simulink model "aerotest"  (R2021b)
settings: Solver=VariableStepAuto  StartTime=0.0  StopTime=10.0  RelTol=1e-3
undefined symbols (not defined in the file or in its folder): admireDB
libraries: simulink_extras x103, simulink x24, aerolibatmos2 x1
(part 1 of 13)
settings Model: Creator=mehme  LastModifiedBy=mehme

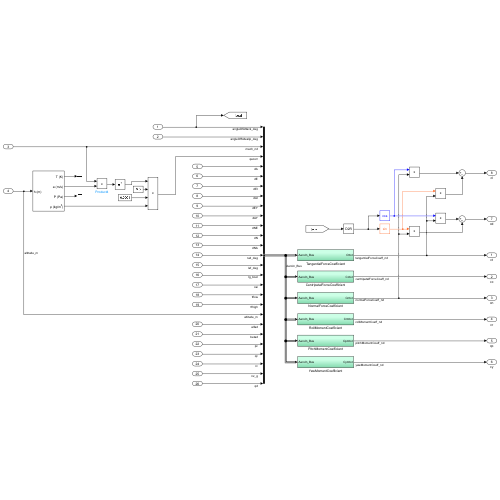
[thumbnail: Simulink's stored preview of the top-level diagram]
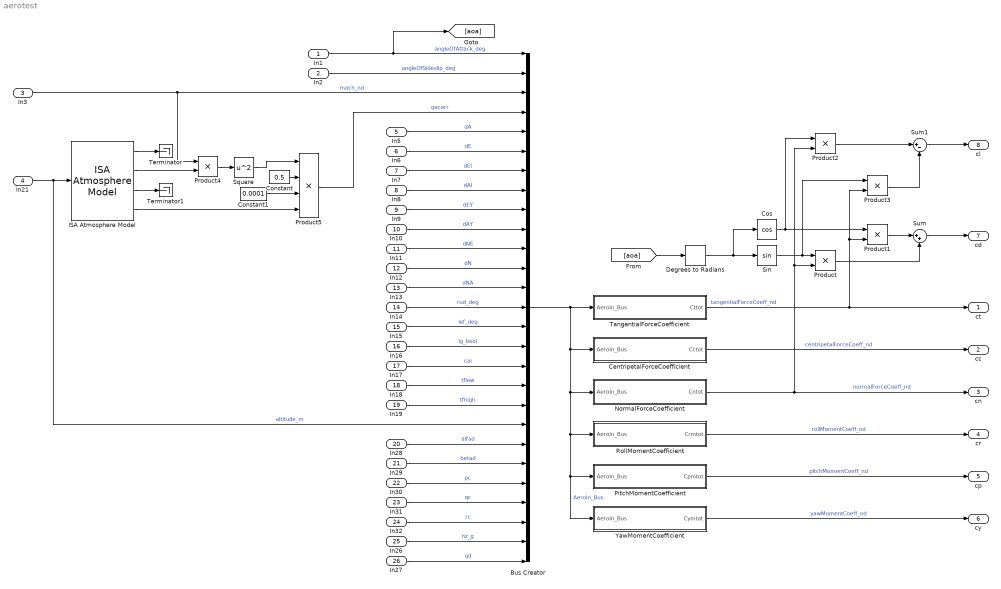
== system aerotest ==
  In1 : Inport
  In2 : Inport  Port=2
  In3 : Inport  Port=3
  In21 : Inport  Port=4
  In5 : Inport  Port=5
  In6 : Inport  Port=6
  In7 : Inport  Port=7
  In8 : Inport  Port=8
  In9 : Inport  Port=9
  In10 : Inport  Port=10
  In11 : Inport  Port=11
  In12 : Inport  Port=12
  In13 : Inport  Port=13
  In14 : Inport  Port=14
  In15 : Inport  Port=15
  In16 : Inport  Port=16
  In17 : Inport  Port=17
  In18 : Inport  Port=18
  In19 : Inport  Port=19
  In28 : Inport  Port=20
  In29 : Inport  Port=21
  In30 : Inport  Port=22
  In31 : Inport  Port=23
  In32 : Inport  Port=24
  In26 : Inport  Port=25
  In27 : Inport  Port=26
  Bus Creator : BusCreator  Inputs=27
  CentripetalForceCoefficient : Subsystem
  Constant : Constant  Value=0.5
  Constant1 : Constant  Value=0.0001
  Cos : Trigonometry  Operator=cos
  Degrees to Radians : simulink_extras/Transformations/Degrees to Radians
  ISA Atmosphere Model : aerolibatmos2/ISA Atmosphere Model  custom=off  g=9.80665  gamma=1.4  R=287.0531  L=0.0065  h_trop=11000  h_strat=20000  rho0=1.225  P0=101325  T0=288.15  h0=0
  NormalForceCoefficient : Subsystem
  PitchMomentCoefficient : Subsystem
  Product{,1..4} (5 alike) : Product
  Product5 : Product  Inputs=4
  RollMomentCoefficient : Subsystem
  Sin : Trigonometry
  Square : Math  Operator=square  SaturateOnIntegerOverflow=on
  Sum : Sum  Inputs=|++
  Sum1 : Sum  Inputs=|+-
  TangentialForceCoefficient : Subsystem
  Terminator : Terminator
  Terminator1 : Terminator
  YawMomentCoefficient : Subsystem
  ct : Outport
  cc : Outport  Port=2
  cn : Outport  Port=3
  cr : Outport  Port=4
  cp : Outport  Port=5
  cy : Outport  Port=6
  cd : Outport  Port=7
  cl : Outport  Port=8
  wires:
  Bus Creator/1 -> TangentialForceCoefficient/1(AeroIn_Bus), CentripetalForceCoefficient/1(AeroIn_Bus), NormalForceCoefficient/1(AeroIn_Bus), RollMomentCoefficient/1(AeroIn_Bus), YawMomentCoefficient/1(AeroIn_Bus), PitchMomentCoefficient/1(AeroIn_Bus)  "AeroIn_Bus"
  CentripetalForceCoefficient/1(Cctot) -> cc/1  "centripetalForceCoeff_nd"
  TangentialForceCoefficient/1(Cttot) -> Product3/2, Product1/2, ct/1  "tangentialForceCoeff_nd"
  NormalForceCoefficient/1(Cntot) -> cn/1, Product2/2, Product/2  "normalForceCoeff_nd"
  YawMomentCoefficient/1(Cymtot) -> cy/1  "yawMomentCoeff_nd"
  RollMomentCoefficient/1(Crmtot) -> cr/1  "rollMomentCoeff_nd"
  PitchMomentCoefficient/1(Cpmtot) -> cp/1  "pitchMomentCoeff_nd"
  In10/1 -> Bus Creator/10  "dAY"
  In16/1 -> Bus Creator/16  "lg_bool"
  In26/1 -> Bus Creator/26  "nz_g"
  In18/1 -> Bus Creator/18  "tflow"
  In14/1 -> Bus Creator/14  "rud_deg"
  In31/1 -> Bus Creator/24  "qc"
  In30/1 -> Bus Creator/23  "pc"
  In28/1 -> Bus Creator/21  "alfad"
  In15/1 -> Bus Creator/15  "lef_deg"
  In7/1 -> Bus Creator/7  "dEI"
  In13/1 -> Bus Creator/13  "dNA"
  In11/1 -> Bus Creator/11  "dNE"
  In21/1 -> Bus Creator/20, ISA Atmosphere Model/1  "altitude_m"
  In8/1 -> Bus Creator/8  "dAI"
  In17/1 -> Bus Creator/17  "cai"
  In5/1 -> Bus Creator/5  "dA"
  In9/1 -> Bus Creator/9  "dEY"
  In19/1 -> Bus Creator/19  "tfhigh"
  In6/1 -> Bus Creator/6  "dE"
  In2/1 -> Bus Creator/2  "angleOfSideslip_deg"
  Product5/1 -> Bus Creator/4  "qacorr"
  In27/1 -> Bus Creator/27  "qd"
  In3/1 -> Bus Creator/3, Product4/1  "mach_nd"
  In12/1 -> Bus Creator/12  "dN"
  In1/1 -> Bus Creator/1, [aoa]  "angleOfAttack_deg"
  In29/1 -> Bus Creator/22  "betad"
  In32/1 -> Bus Creator/25  "rc"
  Degrees to Radians/1 -> Cos/1, Sin/1
  Sin/1 -> Product3/1, Product/1
  Cos/1 -> Product2/1, Product1/1
  Product1/1 -> Sum/1
  Product/1 -> Sum/2
  Product2/1 -> Sum1/1
  Product3/1 -> Sum1/2
  Sum/1 -> cd/1
  Sum1/1 -> cl/1
  ISA Atmosphere Model/1 -> Terminator/1
  ISA Atmosphere Model/3 -> Terminator1/1
  ISA Atmosphere Model/2 -> Product4/2
  Product4/1 -> Square/1
  Square/1 -> Product5/1
  ISA Atmosphere Model/4 -> Product5/4
  Constant/1 -> Product5/2
  Constant1/1 -> Product5/3
  [aoa] -> Degrees to Radians/1

== system aerotest/CentripetalForceCoefficient ==
  AeroIn_Bus : Inport
  Bus Selector : BusSelector  OutputSignals=mach_nd
  MachRegion1 : Subsystem
  MachRegion2 : Subsystem
  MachRegion3 : Subsystem
  MachRegion4 : Subsystem
  Subsystem : Subsystem
  Cctot : Outport
  wires:
  Subsystem/1(Cctot) -> Cctot/1
  MachRegion3/1(cctot) -> Subsystem/4(CctotMR3)
  MachRegion2/1(cctot) -> Subsystem/3(CctotMR2)
  MachRegion4/1(cttot) -> Subsystem/5(CctotMR4)
  Bus Selector/1 -> Subsystem/1(mach_nd)  "<mach_nd>"
  AeroIn_Bus/1 -> MachRegion2/1(AeroIn_Bus), MachRegion3/1(AeroIn_Bus), MachRegion4/1(AeroIn_Bus), MachRegion1/1(AeroIn_Bus), Bus Selector/1
  MachRegion1/1(cctot) -> Subsystem/2(CctotMR1)

== system aerotest/NormalForceCoefficient ==
  AeroIn_Bus : Inport
  Bus Selector : BusSelector  OutputSignals=mach_nd
  MachRegion1 : Subsystem
  MachRegion2 : Subsystem
  MachRegion3 : Subsystem
  Subsystem : Subsystem
  Cntot : Outport
  wires:
  Subsystem/1(Cntot) -> Cntot/1
  Bus Selector/1 -> Subsystem/1(mach_nd)  "<mach_nd>"
  MachRegion2/1(Cntot) -> Subsystem/3(CntotMR2)
  AeroIn_Bus/1 -> MachRegion2/1(Misc_Bus), MachRegion3/1(Misc_Bus), MachRegion1/1(Misc_Bus), Bus Selector/1
  MachRegion3/1(Cntot) -> Subsystem/4(CntotMR3)
  MachRegion1/1(Cntot) -> Subsystem/2(CntotMR1)

== system aerotest/PitchMomentCoefficient ==
  AeroIn_Bus : Inport
  Bus Selector : BusSelector  OutputSignals=mach_nd
  MachRegion1 : Subsystem
  MachRegion2 : Subsystem
  MachRegion3 : Subsystem
  Subsystem : Subsystem
  Cpmtot : Outport
  wires:
  Subsystem/1(Cpmtot) -> Cpmtot/1
  MachRegion1/1(Cpmtot) -> Subsystem/2(CpmtotMR1)
  MachRegion2/1(Cpmtot) -> Subsystem/3(CpmtotMR2)
  MachRegion3/1(Cpmtot) -> Subsystem/4(CpmtotMR3)
  AeroIn_Bus/1 -> MachRegion2/1(Misc_Bus), MachRegion3/1(Misc_Bus), MachRegion1/1(Misc_Bus), Bus Selector/1
  Bus Selector/1 -> Subsystem/1(mach_nd)  "<mach_nd>"

== system aerotest/RollMomentCoefficient ==
  AeroIn_Bus : Inport
  Bus Selector : BusSelector  OutputSignals=mach_nd
  MachRegion1 : Subsystem
  MachRegion2 : Subsystem
  MachRegion3 : Subsystem
  MachRegion4 : Subsystem
  Subsystem : Subsystem
  Crmtot : Outport
  wires:
  Subsystem/1(Crmtot) -> Crmtot/1
  MachRegion4/1(crmtot) -> Subsystem/5(CrmtotMR4)
  MachRegion3/1(crmtot) -> Subsystem/4(CrmtotMR3)
  MachRegion2/1(crmtot) -> Subsystem/3(CrmtotMR2)
  MachRegion1/1(crmtot) -> Subsystem/2(CrmtotMR1)
  Bus Selector/1 -> Subsystem/1(mach_nd)  "<mach_nd>"
  AeroIn_Bus/1 -> MachRegion1/1(AeroIn_Bus), Bus Selector/1, MachRegion2/1(AeroIn_Bus), MachRegion3/1(AeroIn_Bus), MachRegion4/1(AeroIn_Bus)

== system aerotest/TangentialForceCoefficient ==
  AeroIn_Bus : Inport
  Bus Selector : BusSelector  OutputSignals=mach_nd
  MachRegion1 : Subsystem
  MachRegion2 : Subsystem
  MachRegion3 : Subsystem
  Subsystem : Subsystem
  Cttot : Outport
  wires:
  Subsystem/1(Out1) -> Cttot/1
  MachRegion3/1(cttotMR3) -> Subsystem/4(cttotMR3)
  MachRegion2/1(cttotMR2) -> Subsystem/3(cttotMR2)
  MachRegion1/1(cttotMR1) -> Subsystem/2(cttotMR1)
  Bus Selector/1 -> Subsystem/1(mach_nd)  "<mach_nd>"
  AeroIn_Bus/1 -> MachRegion1/1(AeroIn_Bus), MachRegion2/1(AeroIn_Bus), MachRegion3/1(AeroIn_Bus), Bus Selector/1  "AeroIn_Bus"

== system aerotest/YawMomentCoefficient ==
  AeroIn_Bus : Inport
  Bus Selector : BusSelector  OutputSignals=mach_nd
  MachRegion1 : Subsystem
  MachRegion2 : Subsystem
  MachRegion3 : Subsystem
  MachRegion4 : Subsystem
  Subsystem : Subsystem
  Cymtot : Outport
  wires:
  Subsystem/1(Cymtot) -> Cymtot/1
  Bus Selector/1 -> Subsystem/1(mach_nd)  "<mach_nd>"
  MachRegion1/1(Cymtot) -> Subsystem/2(CymtotMR1)
  MachRegion3/1(Cymtot) -> Subsystem/4(CymtotMR3)
  AeroIn_Bus/1 -> MachRegion1/1(AeroIn_Bus), Bus Selector/1, MachRegion2/1(AeroIn_Bus), MachRegion3/1(AeroIn_Bus), MachRegion4/1(AeroIn_Bus)
  MachRegion4/1(Cymtot) -> Subsystem/5(CymtotMR4)
  MachRegion2/1(Cymtot) -> Subsystem/3(CymtotMR2)

== system aerotest/CentripetalForceCoefficient/MachRegion1 ==
  note: Mach <= 0.4
  AeroIn_Bus : Inport
  Bus Creator : BusCreator  Inputs=3
  Ccbcai : Subsystem
  Ccbde : Subsystem
  Ccbdle : Subsystem
  Ccbdn : Subsystem
  Ccbeta : Subsystem
  Ccbetad : Subsystem
  Ccblg : Subsystem
  Ccdai : Subsystem
  Ccdaib : Subsystem
  Ccday : Subsystem
  Ccdayb : Subsystem
  Ccdna : Subsystem
  Ccdr : Subsystem
  Ccp : Subsystem
  Ccpbeta : Subsystem
  Ccr : Subsystem
  Ccrbeta : Subsystem
  Sum : Sum  Inputs=17
  eoeff1 : Subsystem
  cctot : Outport
  wires:
  Ccrbeta/1(Ccrbeta) -> Sum/17  "Ccrbeta"
  Ccr/1(Ccr) -> Sum/16  "Ccr"
  Ccpbeta/1(Ccpbeta) -> Sum/15  "Ccpbeta"
  Ccp/1(Ccp) -> Sum/14  "Ccp"
  Ccbetad/1(Ccbetad) -> Sum/13  "Ccbetad"
  Ccdna/1(Ccdna) -> Sum/12  "Ccdna"
  Ccdayb/1(Ccdayb) -> Sum/11  "Ccdayb"
  Ccday/1(Ccday) -> Sum/10  "Ccday"
  Ccdaib/1(Ccdaib) -> Sum/9  "Ccdaib"
  Ccdai/1(Ccdai) -> Sum/8  "Ccdai"
  Ccdr/1(Ccdr) -> Sum/7  "Ccdr"
  Ccbcai/1(Ccbcai) -> Sum/6  "Ccbcai"
  Ccbdle/1(Ccbdle) -> Sum/5  "Ccbdle"
  Ccbdn/1(Ccbdn) -> Sum/4  "Ccbdn"
  Ccbde/1(Ccbde) -> Sum/3  "Ccbde"
  Ccblg/1(Ccblg) -> Sum/2  "Ccblg"
  Ccbeta/1(Ccbeta) -> Sum/1  "Ccbeta"
  Bus Creator/1 -> Ccp/1(in_bus), Ccpbeta/1(in_bus), Ccr/1(in_bus), Ccrbeta/1(in_bus), Ccbetad/1(in_bus), Ccdna/1(in_bus), Ccdayb/1(in_bus), Ccday/1(in_bus), Ccdaib/1(in_bus), Ccdai/1(in_bus), Ccdr/1(in_bus), Ccbcai/1(in_bus), Ccbdle/1(in_bus), Ccbdn/1(in_bus), Ccbde/1(in_bus), Ccblg/1(in_bus), Ccbeta/1(in_bus)  "in_bus"
  eoeff1/2(eieff) -> Bus Creator/3  "eieff"
  AeroIn_Bus/1 -> eoeff1/1(AeroIn_Bus), Bus Creator/1
  eoeff1/1(eoeff) -> Bus Creator/2  "eoeff"
  Sum/1 -> cctot/1

== system aerotest/CentripetalForceCoefficient/MachRegion2 ==
  note: 0.4 < Mach < 0.5
  AeroIn_Bus : Inport
  Bus Creator : BusCreator  Inputs=3
  Ccbcai : Subsystem
  Ccbde : Subsystem
  Ccbdle : Subsystem
  Ccbdn : Subsystem
  Ccbeta : Subsystem
  Ccbetad : Subsystem
  Ccblg : Subsystem
  Ccdai : Subsystem
  Ccdaib : Subsystem
  Ccday : Subsystem
  Ccdayb : Subsystem
  Ccdna : Subsystem
  Ccdr : Subsystem
  Ccp : Subsystem
  Ccpbeta : Subsystem
  Ccr : Subsystem
  Ccrbeta : Subsystem
  Sum : Sum  Inputs=17
  eoeff1 : Subsystem
  cctot : Outport
  wires:
  Ccrbeta/1(Ccrbeta) -> Sum/17  "Ccrbeta"
  Ccr/1(Ccr) -> Sum/16  "Ccr"
  Ccpbeta/1(Ccpbeta) -> Sum/15  "Ccpbeta"
  Ccp/1(Ccp) -> Sum/14  "Ccp"
  Ccbetad/1(Ccbetad) -> Sum/13  "Ccbetad"
  Ccdna/1(Ccdna) -> Sum/12  "Ccdna"
  Ccdayb/1(Ccdayb) -> Sum/11  "Ccdayb"
  Ccday/1(Ccday) -> Sum/10  "Ccday"
  Ccdaib/1(Ccdaib) -> Sum/9  "Ccdaib"
  Ccdai/1(Ccdai) -> Sum/8  "Ccdai"
  Ccdr/1(Ccdr) -> Sum/7  "Ccdr"
  Ccbcai/1(Ccbcai) -> Sum/6  "Ccbcai"
  Ccbdle/1(Ccbdle) -> Sum/5  "Ccbdle"
  Ccbdn/1(Ccbdn) -> Sum/4  "Ccbdn"
  Ccbde/1(Ccbde) -> Sum/3  "Ccbde"
  Ccblg/1(Ccblg) -> Sum/2  "Ccblg"
  Ccbeta/1(Ccbeta) -> Sum/1  "Ccbeta"
  Bus Creator/1 -> Ccr/1(in_bus), Ccrbeta/1(in_bus), Ccpbeta/1(in_bus), Ccp/1(in_bus), Ccbetad/1(in_bus), Ccdna/1(in_bus), Ccdayb/1(in_bus), Ccday/1(in_bus), Ccdaib/1(in_bus), Ccdai/1(in_bus), Ccdr/1(in_bus), Ccbcai/1(in_bus), Ccbdle/1(in_bus), Ccbdn/1(in_bus), Ccbde/1(in_bus), Ccblg/1(in_bus), Ccbeta/1(in_bus)  "in_bus"
  eoeff1/1(eoeff) -> Bus Creator/2  "eoeff"
  eoeff1/2(eieff) -> Bus Creator/3  "eieff"
  AeroIn_Bus/1 -> eoeff1/1(AeroIn_Bus), Bus Creator/1
  Sum/1 -> cctot/1

== system aerotest/CentripetalForceCoefficient/MachRegion3 ==
  note: 0.5 <= Mach <= 1.4
  AeroIn_Bus : Inport
  Bus Creator : BusCreator  Inputs=3
  Ccbcai : Subsystem
  Ccbde : Subsystem
  Ccbdle : Subsystem
  Ccbdn : Subsystem
  Ccbeta : Subsystem
  Ccbetad : Subsystem
  Ccblg : Subsystem
  Ccdai : Subsystem
  Ccdaib : Subsystem
  Ccday : Subsystem
  Ccdayb : Subsystem
  Ccdna : Subsystem
  Ccdr : Subsystem
  Ccp1 : Subsystem
  Ccpbeta : Subsystem
  Ccr1 : Subsystem
  Ccrbeta : Subsystem
  Sum : Sum  Inputs=17
  eoeff1 : Subsystem
  cctot : Outport
  wires:
  Ccrbeta/1(Ccrbeta) -> Sum/17  "Ccrbeta"
  Ccr1/1(Ccr) -> Sum/16  "Ccr"
  Ccpbeta/1(Ccpbeta) -> Sum/15  "Ccpbeta"
  Ccp1/1(Ccp) -> Sum/14  "Ccp"
  Ccbetad/1(Ccbetad) -> Sum/13  "Ccbetad"
  Ccdna/1(Ccdna) -> Sum/12  "Ccdna"
  Ccdayb/1(Ccdayb) -> Sum/11  "Ccdayb"
  Ccday/1(Ccday) -> Sum/10  "Ccday"
  Ccdaib/1(Ccdaib) -> Sum/9  "Ccdaib"
  Ccdai/1(Ccdai) -> Sum/8  "Ccdai"
  Ccdr/1(Ccdr) -> Sum/7  "Ccdr"
  Ccbcai/1(Ccbcai) -> Sum/6  "Ccbcai"
  Ccbdle/1(Ccbdle) -> Sum/5  "Ccbdle"
  Ccbdn/1(Ccbdn) -> Sum/4  "Ccbdn"
  Ccbde/1(Ccbde) -> Sum/3  "Ccbde"
  Ccblg/1(Ccblg) -> Sum/2  "Ccblg"
  Ccbeta/1(Ccbeta) -> Sum/1  "Ccbeta"
  eoeff1/2(eieff) -> Bus Creator/3  "eieff"
  eoeff1/1(eoeff) -> Bus Creator/2  "eoeff"
  Bus Creator/1 -> Ccr1/1(in_bus), Ccp1/1(in_bus), Ccbetad/1(in_bus), Ccdna/1(in_bus), Ccday/1(in_bus), Ccdai/1(in_bus), Ccdr/1(in_bus), Ccbcai/1(in_bus), Ccbdle/1(in_bus), Ccbdn/1(in_bus), Ccbde/1(in_bus), Ccblg/1(in_bus), Ccbeta/1(in_bus)  "in_bus"
  AeroIn_Bus/1 -> eoeff1/1(AeroIn_Bus), Bus Creator/1
  Sum/1 -> cctot/1

== system aerotest/CentripetalForceCoefficient/MachRegion4 ==
  note: 1.4 < Mach
  AeroIn_Bus : Inport
  Bus Creator : BusCreator  Inputs=3
  Ccbcai : Subsystem
  Ccbde : Subsystem
  Ccbdle : Subsystem
  Ccbdn : Subsystem
  Ccbeta : Subsystem
  Ccbetad : Subsystem
  Ccblg : Subsystem
  Ccdai : Subsystem
  Ccdaib : Subsystem
  Ccday : Subsystem
  Ccdayb : Subsystem
  Ccdna : Subsystem
  Ccdr : Subsystem
  Ccp : Subsystem
  Ccpbeta : Subsystem
  Ccr : Subsystem
  Ccrbeta : Subsystem
  Sum : Sum  Inputs=17
  eoeff : Subsystem
  cttot : Outport
  wires:
  Ccrbeta/1(Ccrbeta) -> Sum/17  "Ccrbeta"
  Ccr/1(Ccr) -> Sum/16  "Ccr"
  Ccpbeta/1(Ccpbeta) -> Sum/15  "Ccpbeta"
  Ccp/1(Ccp) -> Sum/14  "Ccp"
  Ccbetad/1(Ccbetad) -> Sum/13  "Ccbetad"
  Ccdna/1(Ccdna) -> Sum/12  "Ccdna"
  Ccdayb/1(Ccdayb) -> Sum/11  "Ccdayb"
  Ccday/1(Ccday) -> Sum/10  "Ccday"
  Ccdaib/1(Ccdaib) -> Sum/9  "Ccdaib"
  Ccdai/1(Ccdai) -> Sum/8  "Ccdai"
  Ccblg/1(Ccblg) -> Sum/7  "Ccblg"
  Ccdr/1(Ccdr) -> Sum/6  "Ccdr"
  Ccbcai/1(Ccbcai) -> Sum/5  "Ccbcai"
  Ccbdle/1(Ccbdle) -> Sum/4  "Ccbdle"
  Ccbdn/1(Ccbdn) -> Sum/3  "Ccbdn"
  Ccbde/1(Ccbde) -> Sum/2  "Ccbde"
  Ccbeta/1(Ccbeta) -> Sum/1  "Ccbeta"
  AeroIn_Bus/1 -> eoeff/1(AeroIn_Bus), Bus Creator/1
  Bus Creator/1 -> Ccbde/1(in_bus), Ccbdn/1(in_bus), Ccbdle/1(in_bus), Ccbcai/1(in_bus), Ccdr/1(in_bus), Ccr/1(in_bus), Ccp/1(in_bus), Ccbetad/1(in_bus), Ccdna/1(in_bus), Ccday/1(in_bus), Ccdai/1(in_bus), Ccblg/1(in_bus), Ccbeta/1(in_bus)  "in_bus"
  eoeff/2(eieff) -> Bus Creator/3  "eieff"
  eoeff/1(eoeff) -> Bus Creator/2  "eoeff"
  Sum/1 -> cttot/1

== system aerotest/CentripetalForceCoefficient/Subsystem ==
  mach_nd : Inport
  CctotMR1 : Inport  Port=2
  CctotMR2 : Inport  Port=3
  CctotMR3 : Inport  Port=4
  CctotMR4 : Inport  Port=5
  AND : Logic  IconShape=distinctive  AllPortsSameDT=off  OutDataTypeStr=boolean
  AND1 : Logic  IconShape=distinctive  AllPortsSameDT=off  OutDataTypeStr=boolean
  Compare To Constant1 : simulink/Logic and Bit Operations/Compare To Constant  relop=<=  const=0.4  OutDataTypeStr=boolean
  Compare To Constant2 : simulink/Logic and Bit Operations/Compare To Constant  relop=>  const=0.4  OutDataTypeStr=boolean
  Compare To Constant3 : simulink/Logic and Bit Operations/Compare To Constant  relop=<  const=0.5  OutDataTypeStr=boolean
  Compare To Constant4 : simulink/Logic and Bit Operations/Compare To Constant  relop=<=  const=1.4  OutDataTypeStr=boolean
  Compare To Constant5 : simulink/Logic and Bit Operations/Compare To Constant  relop=>=  const=0.5  OutDataTypeStr=boolean
  Switch : Switch  Criteria=u2 ~= 0
  Switch1 : Switch  Criteria=u2 ~= 0
  Switch2 : Switch  Criteria=u2 ~= 0
  Cctot : Outport
  wires:
  Switch/1 -> Cctot/1
  Compare To Constant5/1 -> AND1/1
  Compare To Constant4/1 -> AND1/2
  AND1/1 -> Switch2/2
  CctotMR4/1 -> Switch2/3
  CctotMR3/1 -> Switch2/1
  CctotMR1/1 -> Switch/1
  Switch2/1 -> Switch1/3
  CctotMR2/1 -> Switch1/1
  Switch1/1 -> Switch/3
  AND/1 -> Switch1/2
  Compare To Constant3/1 -> AND/2
  Compare To Constant2/1 -> AND/1
  Compare To Constant1/1 -> Switch/2
  mach_nd/1 -> Compare To Constant1/1, Compare To Constant3/1, Compare To Constant4/1, Compare To Constant5/1, Compare To Constant2/1

== system aerotest/NormalForceCoefficient/MachRegion1 ==
  note: Mach <= 0.4
  Misc_Bus : Inport
  Bus Creator : BusCreator  Inputs=3
  Cnalfa : Subsystem
  Cnalfad : Subsystem
  Cnbasic : Subsystem
  Cnbeta : Subsystem
  Cncai : Subsystem
  Cndedn : Subsystem
  Cndei : Subsystem
  Cndey : Subsystem
  Cndle : Subsystem
  Cndn : Subsystem
  Cnhigh : Subsystem
  Cnlg : Subsystem
  Cnnz : Subsystem
  Cnq : Subsystem
  Cnqd : Subsystem
  Sum : Sum  Inputs=15
  eoeff : Subsystem
  Cntot : Outport
  wires:
  Sum/1 -> Cntot/1
  Cnhigh/1(Cnhigh) -> Sum/15  "Cnhigh"
  Cnqd/1(Cnqd) -> Sum/14  "Cnqd"
  Cnnz/1(Cnnz) -> Sum/13  "Cnnz"
  Cnq/1(Cnq) -> Sum/12  "Cnq"
  Cnalfad/1(Cnalfad) -> Sum/11  "Cnalfad"
  Cnlg/1(Cnlg) -> Sum/10  "Cnlg"
  Cnbeta/1(Cnbeta) -> Sum/9  "Cnbeta"
  Cncai/1(Cncai) -> Sum/8  "Cncai"
  Cndle/1(Cndle) -> Sum/7  "Cndle"
  Cndn/1(Cndn) -> Sum/6  "Cndn"
  Cndedn/1(Cndedn) -> Sum/5  "Cndedn"
  Cndey/1(Cndey) -> Sum/4  "Cndey"
  Cndei/1(Cndei) -> Sum/3  "Cndei"
  Cnalfa/1(Cnalfa) -> Sum/2  "Cnalfa"
  Cnbasic/1(Cnbasic) -> Sum/1  "Cnbasic"
  Bus Creator/1 -> Cnbasic/1(in_bus), Cnalfa/1(in_bus), Cndei/1(in_bus), Cndey/1(in_bus), Cndedn/1(in_bus), Cndn/1(in_bus), Cndle/1(in_bus), Cncai/1(in_bus), Cnbeta/1(in_bus), Cnlg/1(in_bus), Cnalfad/1(in_bus), Cnq/1(in_bus), Cnnz/1(in_bus), Cnqd/1(in_bus), Cnhigh/1(in_bus)  "in_bus"
  eoeff/1(eoeff) -> Bus Creator/2  "eoeff"
  Misc_Bus/1 -> eoeff/1(AeroIn_Bus), Bus Creator/1
  eoeff/2(eieff) -> Bus Creator/3  "eieff"

== system aerotest/NormalForceCoefficient/MachRegion2 ==
  note: 0.4 < Mach < 0.5
  Misc_Bus : Inport
  Bus Creator : BusCreator  Inputs=3
  Cnalfa : Subsystem
  Cnalfad : Subsystem
  Cnbasic : Subsystem
  Cnbeta : Subsystem
  Cncai : Subsystem
  Cndedn : Subsystem
  Cndei : Subsystem
  Cndey : Subsystem
  Cndle : Subsystem
  Cndn : Subsystem
  Cnhigh : Subsystem
  Cnlg : Subsystem
  Cnnz : Subsystem
  Cnq : Subsystem
  Cnqd : Subsystem
  Sum : Sum  Inputs=15
  eoeff : Subsystem
  Cntot : Outport
  wires:
  Sum/1 -> Cntot/1
  eoeff/2(eieff) -> Bus Creator/3  "eieff"
  Misc_Bus/1 -> Bus Creator/1, eoeff/1(AeroIn_Bus)
  eoeff/1(eoeff) -> Bus Creator/2  "eoeff"
  Bus Creator/1 -> Cnqd/1(in_bus), Cnnz/1(in_bus), Cnq/1(in_bus), Cnalfad/1(in_bus), Cnlg/1(in_bus), Cnbeta/1(in_bus), Cncai/1(in_bus), Cndle/1(in_bus), Cndn/1(in_bus), Cndedn/1(in_bus), Cndey/1(in_bus), Cndei/1(in_bus), Cnalfa/1(in_bus), Cnbasic/1(in_bus)  "in_bus"
  Cnbasic/1(Cnbasic) -> Sum/1  "Cnbasic"
  Cnalfa/1(Cnalfa) -> Sum/2  "Cnalfa"
  Cndei/1(Cndei) -> Sum/3  "Cndei"
  Cndey/1(Cndey) -> Sum/4  "Cndey"
  Cndedn/1(Cndedn) -> Sum/5  "Cndedn"
  Cndn/1(Cndn) -> Sum/6  "Cndn"
  Cndle/1(Cndle) -> Sum/7  "Cndle"
  Cncai/1(Cncai) -> Sum/8  "Cncai"
  Cnbeta/1(Cnbeta) -> Sum/9  "Cnbeta"
  Cnlg/1(Cnlg) -> Sum/10  "Cnlg"
  Cnalfad/1(Cnalfad) -> Sum/11  "Cnalfad"
  Cnq/1(Cnq) -> Sum/12  "Cnq"
  Cnnz/1(Cnnz) -> Sum/13  "Cnnz"
  Cnqd/1(Cnqd) -> Sum/14  "Cnqd"
  Cnhigh/1(Cnhigh) -> Sum/15  "Cnhigh"

== system aerotest/NormalForceCoefficient/MachRegion3 ==
  note: 0.5 <= Mach
  Misc_Bus : Inport
  Bus Creator : BusCreator  Inputs=3
  Cnalfa : Subsystem
  Cnalfad : Subsystem
  Cnbasic : Subsystem
  Cnbeta : Subsystem
  Cncai : Subsystem
  Cndedn : Subsystem
  Cndei : Subsystem
  Cndey : Subsystem
  Cndle : Subsystem
  Cndn : Subsystem
  Cnhigh : Subsystem
  Cnlg : Subsystem
  Cnnz : Subsystem
  Cnq : Subsystem
  Cnqd : Subsystem
  Sum : Sum  Inputs=15
  eoeff : Subsystem
  Cntot : Outport
  wires:
  Sum/1 -> Cntot/1
  eoeff/2(eieff) -> Bus Creator/3  "eieff"
  Misc_Bus/1 -> Bus Creator/1, eoeff/1(AeroIn_Bus)
  eoeff/1(eoeff) -> Bus Creator/2  "eoeff"
  Bus Creator/1 -> Cnqd/1(in_bus), Cnnz/1(in_bus), Cnq/1(in_bus), Cnalfad/1(in_bus), Cnlg/1(in_bus), Cncai/1(in_bus), Cndle/1(in_bus), Cndn/1(in_bus), Cndey/1(in_bus), Cndei/1(in_bus), Cnalfa/1(in_bus), Cnbasic/1(in_bus)  "in_bus"
  Cnbasic/1(Cnbasic) -> Sum/1  "Cnbasic"
  Cnalfa/1(Cnalfa) -> Sum/2  "Cnalfa"
  Cndei/1(Cndei) -> Sum/3  "Cndei"
  Cndey/1(Cndey) -> Sum/4  "Cndey"
  Cndedn/1(Cndedn) -> Sum/5  "Cndedn"
  Cndn/1(Cndn) -> Sum/6  "Cndn"
  Cndle/1(Cndle) -> Sum/7  "Cndle"
  Cncai/1(Cncai) -> Sum/8  "Cncai"
  Cnbeta/1(Cnbeta) -> Sum/9  "Cnbeta"
  Cnlg/1(Cnlg) -> Sum/10  "Cnlg"
  Cnalfad/1(Cnalfad) -> Sum/11  "Cnalfad"
  Cnq/1(Cnq) -> Sum/12  "Cnq"
  Cnnz/1(Cnnz) -> Sum/13  "Cnnz"
  Cnqd/1(Cnqd) -> Sum/14  "Cnqd"
  Cnhigh/1(Cnhigh) -> Sum/15  "Cnhigh"

== system aerotest/NormalForceCoefficient/Subsystem ==
  mach_nd : Inport
  CntotMR1 : Inport  Port=2
  CntotMR2 : Inport  Port=3
  CntotMR3 : Inport  Port=4
  AND : Logic  IconShape=distinctive  AllPortsSameDT=off  OutDataTypeStr=boolean
  Compare To Constant1 : simulink/Logic and Bit Operations/Compare To Constant  relop=<=  const=0.4  OutDataTypeStr=boolean
  Compare To Constant2 : simulink/Logic and Bit Operations/Compare To Constant  relop=>  const=0.4  OutDataTypeStr=boolean
  Compare To Constant3 : simulink/Logic and Bit Operations/Compare To Constant  relop=<  const=0.5  OutDataTypeStr=boolean
  Switch : Switch  Criteria=u2 ~= 0
  Switch1 : Switch  Criteria=u2 ~= 0
  Cntot : Outport
  wires:
  Switch/1 -> Cntot/1
  CntotMR3/1 -> Switch1/3
  CntotMR2/1 -> Switch1/1
  Switch1/1 -> Switch/3
  CntotMR1/1 -> Switch/1
  AND/1 -> Switch1/2
  Compare To Constant3/1 -> AND/2
  Compare To Constant2/1 -> AND/1
  Compare To Constant1/1 -> Switch/2
  mach_nd/1 -> Compare To Constant1/1, Compare To Constant3/1, Compare To Constant2/1

== system aerotest/PitchMomentCoefficient/MachRegion1 ==
  note: Mach <= 0.4
  Misc_Bus : Inport
  Bus Creator : BusCreator  Inputs=3
  Cpmalfa : Subsystem
  Cpmalfad : Subsystem
  Cpmbasic : Subsystem
  Cpmbeta : Subsystem
  Cpmcai : Subsystem
  Cpmda : Subsystem
  Cpmdedn : Subsystem
  Cpmdei : Subsystem
  Cpmdey : Subsystem
  Cpmdle : Subsystem
  Cpmdn : Subsystem
  Cpmhigh : Subsystem
  Cpmlg : Subsystem
  Cpmnz : Subsystem
  Cpmq : Subsystem
  Cpmqd : Subsystem
  Sum : Sum  Inputs=16
  eoeff : Subsystem
  Cpmtot : Outport
  wires:
  Cpmhigh/1(Cpmhigh) -> Sum/16  "Cpmhigh"
  Cpmqd/1(Cpmqd) -> Sum/15  "Cpmqd"
  Cpmnz/1(Cpmnz) -> Sum/14  "Cpmnz"
  Cpmq/1(Cpmq) -> Sum/13  "Cpmq"
  Cpmalfad/1(Cpmalfad) -> Sum/12  "Cpmalfad"
  Cpmda/1(Cpmda) -> Sum/11  "Cpmda"
  Cpmbasic/1(Cpmbasic) -> Sum/1  "Cpmbasic"
  Cpmbeta/1(Cpmbeta) -> Sum/10  "Cpmbeta"
  Cpmalfa/1(Cpmalfa) -> Sum/2  "Cpmalfa"
  Cpmcai/1(Cpmcai) -> Sum/9  "Cpmcai"
  Cpmdei/1(Cpmdei) -> Sum/3  "Cpmdei"
  Cpmlg/1(Cpmlg) -> Sum/8  "Cpmlg"
  Cpmdey/1(Cpmdey) -> Sum/4  "Cpmdey"
  Cpmdle/1(Cpmdle) -> Sum/7  "Cpmdle"
  Cpmdedn/1(Cpmdedn) -> Sum/5  "Cpmdedn"
  Cpmdn/1(Cpmdn) -> Sum/6  "Cpmdn"
  Bus Creator/1 -> Cpmbasic/1(in_bus), Cpmnz/1(in_bus), Cpmqd/1(in_bus), Cpmhigh/1(in_bus), Cpmq/1(in_bus), Cpmalfad/1(in_bus), Cpmda/1(in_bus), Cpmbeta/1(in_bus), Cpmcai/1(in_bus), Cpmlg/1(in_bus), Cpmdle/1(in_bus), Cpmdn/1(in_bus), Cpmdedn/1(in_bus), Cpmdey/1(in_bus), Cpmdei/1(in_bus), Cpmalfa/1(in_bus)  "in_bus"
  eoeff/1(eoeff) -> Bus Creator/2  "eoeff"
  eoeff/2(eieff) -> Bus Creator/3  "eieff"
  Misc_Bus/1 -> eoeff/1(AeroIn_Bus), Bus Creator/1
  Sum/1 -> Cpmtot/1

== system aerotest/PitchMomentCoefficient/MachRegion2 ==
  note: 0.4 < Mach < 0.5
  Misc_Bus : Inport
  Bus Creator : BusCreator  Inputs=5
  Cpmalfa : Subsystem
  Cpmalfad : Subsystem
  Cpmbasic : Subsystem
  Cpmbeta : Subsystem
  Cpmcai : Subsystem
  Cpmda : Subsystem
  Cpmdedn : Subsystem
  Cpmdei : Subsystem
  Cpmdey : Subsystem
  Cpmdle : Subsystem
  Cpmdn : Subsystem
  Cpmhigh : Subsystem
  Cpmlg : Subsystem
  Cpmnz : Subsystem
  Cpmq : Subsystem
  Cpmqd : Subsystem
  Sum : Sum  Inputs=16
  eoeff : Subsystem
  Cpmtot : Outport
  wires:
  eoeff/3(eoefflow) -> Bus Creator/4  "eoefflow"
  eoeff/4(eiefflow) -> Bus Creator/5  "eiefflow"
  Sum/1 -> Cpmtot/1
  Misc_Bus/1 -> Bus Creator/1, eoeff/1(AeroIn_Bus)
  eoeff/2(eieff) -> Bus Creator/3  "eieff"
  eoeff/1(eoeff) -> Bus Creator/2  "eoeff"
  Bus Creator/1 -> Cpmalfa/1(in_bus), Cpmdei/1(in_bus), Cpmdedn/1(in_bus), Cpmdn/1(in_bus), Cpmdle/1(in_bus), Cpmlg/1(in_bus), Cpmcai/1(in_bus), Cpmbeta/1(in_bus), Cpmda/1(in_bus), Cpmalfad/1(in_bus), Cpmq/1(in_bus), Cpmqd/1(in_bus), Cpmnz/1(in_bus), Cpmdey/1(in_bus), Cpmbasic/1(in_bus)  "in_bus"
  Cpmdn/1(Cpmdn) -> Sum/6  "Cpmdn"
  Cpmdedn/1(Cpmdedn) -> Sum/5  "Cpmdedn"
  Cpmdle/1(Cpmdle) -> Sum/7  "Cpmdle"
  Cpmdey/1(Cpmdey) -> Sum/4  "Cpmdey"
  Cpmlg/1(Cpmlg) -> Sum/8  "Cpmlg"
  Cpmdei/1(Cpmdei) -> Sum/3  "Cpmdei"
  Cpmcai/1(Cpmcai) -> Sum/9  "Cpmcai"
  Cpmalfa/1(Cpmalfa) -> Sum/2  "Cpmalfa"
  Cpmbeta/1(Cpmbeta) -> Sum/10  "Cpmbeta"
  Cpmbasic/1(Cpmbasic) -> Sum/1  "Cpmbasic"
  Cpmda/1(Cpmda) -> Sum/11  "Cpmda"
  Cpmalfad/1(Cpmalfad) -> Sum/12  "Cpmalfad"
  Cpmq/1(Cpmq) -> Sum/13  "Cpmq"
  Cpmnz/1(Cpmnz) -> Sum/14  "Cpmnz"
  Cpmqd/1(Cpmqd) -> Sum/15  "Cpmqd"
  Cpmhigh/1(Cpmhigh) -> Sum/16  "Cpmhigh"

== system aerotest/PitchMomentCoefficient/MachRegion3 ==
  note: 0.5 <= Mach
  Misc_Bus : Inport
  Bus Creator : BusCreator  Inputs=3
  Cpmalfa : Subsystem
  Cpmalfad : Subsystem
  Cpmbasic : Subsystem
  Cpmbeta : Subsystem
  Cpmcai : Subsystem
  Cpmda : Subsystem
  Cpmdedn : Subsystem
  Cpmdei : Subsystem
  Cpmdey : Subsystem
  Cpmdle : Subsystem
  Cpmdn : Subsystem
  Cpmhigh : Subsystem
  Cpmlg : Subsystem
  Cpmnz : Subsystem
  Cpmq : Subsystem
  Cpmqd : Subsystem
  Sum : Sum  Inputs=16
  eoeff : Subsystem
  Cpmtot : Outport
  wires:
  Sum/1 -> Cpmtot/1
  Misc_Bus/1 -> Bus Creator/1, eoeff/1(AeroIn_Bus)
  eoeff/2(eieff) -> Bus Creator/3  "eieff"
  eoeff/1(eoeff) -> Bus Creator/2  "eoeff"
  Bus Creator/1 -> Cpmalfa/1(in_bus), Cpmdei/1(in_bus), Cpmdn/1(in_bus), Cpmdle/1(in_bus), Cpmlg/1(in_bus), Cpmcai/1(in_bus), Cpmalfad/1(in_bus), Cpmq/1(in_bus), Cpmqd/1(in_bus), Cpmnz/1(in_bus), Cpmdey/1(in_bus), Cpmbasic/1(in_bus)  "in_bus"
  Cpmdn/1(Cpmdn) -> Sum/6  "Cpmdn"
  Cpmdedn/1(Cpmdedn) -> Sum/5  "Cpmdedn"
  Cpmdle/1(Cpmdle) -> Sum/7  "Cpmdle"
  Cpmdey/1(Cpmdey) -> Sum/4  "Cpmdey"
  Cpmlg/1(Cpmlg) -> Sum/8  "Cpmlg"
  Cpmdei/1(Cpmdei) -> Sum/3  "Cpmdei"
  Cpmcai/1(Cpmcai) -> Sum/9  "Cpmcai"
  Cpmalfa/1(Cpmalfa) -> Sum/2  "Cpmalfa"
  Cpmbeta/1(Cpmbeta) -> Sum/10  "Cpmbeta"
  Cpmbasic/1(Cpmbasic) -> Sum/1  "Cpmbasic"
  Cpmda/1(Cpmda) -> Sum/11  "Cpmda"
  Cpmalfad/1(Cpmalfad) -> Sum/12  "Cpmalfad"
  Cpmq/1(Cpmq) -> Sum/13  "Cpmq"
  Cpmnz/1(Cpmnz) -> Sum/14  "Cpmnz"
  Cpmqd/1(Cpmqd) -> Sum/15  "Cpmqd"
  Cpmhigh/1(Cpmhigh) -> Sum/16  "Cpmhigh"

== system aerotest/PitchMomentCoefficient/Subsystem ==
  mach_nd : Inport
  CpmtotMR1 : Inport  Port=2
  CpmtotMR2 : Inport  Port=3
  CpmtotMR3 : Inport  Port=4
  AND : Logic  IconShape=distinctive  AllPortsSameDT=off  OutDataTypeStr=boolean
  Compare To Constant1 : simulink/Logic and Bit Operations/Compare To Constant  relop=<=  const=0.4  OutDataTypeStr=boolean
  Compare To Constant2 : simulink/Logic and Bit Operations/Compare To Constant  relop=>  const=0.4  OutDataTypeStr=boolean
  Compare To Constant3 : simulink/Logic and Bit Operations/Compare To Constant  relop=<  const=0.5  OutDataTypeStr=boolean
  Switch : Switch  Criteria=u2 ~= 0
  Switch1 : Switch  Criteria=u2 ~= 0
  Cpmtot : Outport
  wires:
  Switch/1 -> Cpmtot/1
  CpmtotMR3/1 -> Switch1/3
  CpmtotMR2/1 -> Switch1/1
  Switch1/1 -> Switch/3
  CpmtotMR1/1 -> Switch/1
  AND/1 -> Switch1/2
  Compare To Constant3/1 -> AND/2
  Compare To Constant2/1 -> AND/1
  Compare To Constant1/1 -> Switch/2
  mach_nd/1 -> Compare To Constant1/1, Compare To Constant3/1, Compare To Constant2/1

== system aerotest/RollMomentCoefficient/MachRegion1 ==
  note: Mach <= 0.4
  AeroIn_Bus : Inport
  Bus Creator : BusCreator  Inputs=3
  Crmbasic : Subsystem
  Crmbde : Subsystem
  Crmbdle : Subsystem
  Crmbdn : Subsystem
  Crmbeta : Subsystem
  Crmbetad : Subsystem
  Crmblg : Subsystem
  Crmdai : Subsystem
  Crmdaib : Subsystem
  Crmday : Subsystem
  Crmdayb : Subsystem
  Crmdna : Subsystem
  Crmdr : Subsystem
  Crmp : Subsystem
  Crmpbeta : Subsystem
  Crmr : Subsystem
  Crmrbeta : Subsystem
  Crmrde : Subsystem
  Sum : Sum  Inputs=18
  eoeff1 : Subsystem
  crmtot : Outport
  wires:
  Crmrde/1(Crmrbeta) -> Sum/18  "Crmrde"
  Crmrbeta/1(Crmrbeta) -> Sum/17  "Crmrbeta"
  Crmr/1(Crmr) -> Sum/16  "Crmr"
  Crmpbeta/1(Crmpbeta) -> Sum/15  "Crmpbeta"
  Crmp/1(Crmp) -> Sum/14  "Crmp"
  Crmbetad/1(Crmbetad) -> Sum/13  "Crmbetad"
  Crmdna/1(Crmdna) -> Sum/12  "Crmdna"
  Crmdayb/1(Crmdayb) -> Sum/11  "Crmdayb"
  Crmday/1(Crmday) -> Sum/10  "Crmday"
  Crmdaib/1(Crmdaib) -> Sum/9  "Crmdaib"
  Crmdai/1(Crmdai) -> Sum/8  "Crmdai"
  Crmdr/1(Crmdr) -> Sum/7  "Crmdr"
  Crmblg/1(Crmblg) -> Sum/6  "Crmblg"
  Crmbdle/1(Crmbdle) -> Sum/5  "Crmbdle"
  Crmbdn/1(Crmbdn) -> Sum/4  "Crmbdn"
  Crmbde/1(Crmbde) -> Sum/3  "Crmbde"
  Crmbeta/1(Crmbeta) -> Sum/2  "Crmbeta"
  Crmbasic/1(Crmbasic) -> Sum/1  "Crmbasic"
  eoeff1/1(eoeff) -> Bus Creator/2  "eoeff"
  Bus Creator/1 -> Crmr/1(in_bus), Crmrbeta/1(in_bus), Crmrde/1(in_bus), Crmpbeta/1(in_bus), Crmp/1(in_bus), Crmbetad/1(in_bus), Crmdna/1(in_bus), Crmdayb/1(in_bus), Crmday/1(in_bus), Crmdaib/1(in_bus), Crmdai/1(in_bus), Crmdr/1(in_bus), Crmblg/1(in_bus), Crmbdle/1(in_bus), Crmbdn/1(in_bus), Crmbde/1(in_bus), Crmbeta/1(in_bus), Crmbasic/1(in_bus)  "in_bus"
  AeroIn_Bus/1 -> eoeff1/1(AeroIn_Bus), Bus Creator/1
  eoeff1/2(eieff) -> Bus Creator/3  "eieff"
  Sum/1 -> crmtot/1

== system aerotest/RollMomentCoefficient/MachRegion2 ==
  note: 0.4 < Mach < 0.5
  AeroIn_Bus : Inport
  Bus Creator : BusCreator  Inputs=3
  Crmbasic : Subsystem
  Crmbde : Subsystem
  Crmbdle : Subsystem
  Crmbdn : Subsystem
  Crmbeta : Subsystem
  Crmbetad : Subsystem
  Crmblg : Subsystem
  Crmdai : Subsystem
  Crmdaib : Subsystem
  Crmday : Subsystem
  Crmdayb : Subsystem
  Crmdna : Subsystem
  Crmdr : Subsystem
  Crmp : Subsystem
  Crmpbeta : Subsystem
  Crmr : Subsystem
  Crmrbeta : Subsystem
  Crmrde : Subsystem
  Sum : Sum  Inputs=18
  eoeff1 : Subsystem
  crmtot : Outport
  wires:
  Crmpbeta/1(Crmpbeta) -> Sum/15  "Crmpbeta"
  Crmdaib/1(Crmdaib) -> Sum/9  "Crmdaib"
  Crmdai/1(Crmdai) -> Sum/8  "Crmdai"
  Crmbasic/1(Crmbasic) -> Sum/1  "Crmbasic"
  Crmrbeta/1(Crmrbeta) -> Sum/17  "Crmrbeta"
  Crmr/1(Crmr) -> Sum/16  "Crmr"
  Crmdna/1(Crmdna) -> Sum/12  "Crmdna"
  Sum/1 -> crmtot/1
  Crmbetad/1(Crmbetad) -> Sum/13  "Crmbetad"
  Crmp/1(Crmp) -> Sum/14  "Crmp"
  AeroIn_Bus/1 -> eoeff1/1(AeroIn_Bus), Bus Creator/1
  Crmdayb/1(Crmdayb) -> Sum/11  "Crmdayb"
  eoeff1/2(eieff) -> Bus Creator/3  "eieff"
  Crmdr/1(Crmdr) -> Sum/7  "Crmdr"
  Crmbdn/1(Crmbdn) -> Sum/4  "Crmbdn"
  Crmbde/1(Crmbde) -> Sum/3  "Crmbde"
  eoeff1/1(eoeff) -> Bus Creator/2  "eoeff"
  Bus Creator/1 -> Crmr/1(in_bus), Crmrbeta/1(in_bus), Crmrde/1(in_bus), Crmpbeta/1(in_bus), Crmp/1(in_bus), Crmbetad/1(in_bus), Crmdna/1(in_bus), Crmdayb/1(in_bus), Crmday/1(in_bus), Crmdaib/1(in_bus), Crmdai/1(in_bus), Crmdr/1(in_bus), Crmblg/1(in_bus), Crmbdle/1(in_bus), Crmbdn/1(in_bus), Crmbde/1(in_bus), Crmbeta/1(in_bus), Crmbasic/1(in_bus)  "in_bus"
  Crmbdle/1(Crmbdle) -> Sum/5  "Crmbdle"
  Crmday/1(Crmday) -> Sum/10  "Crmday"
  Crmblg/1(Crmblg) -> Sum/6  "Crmblg"
  Crmbeta/1(Crmbeta) -> Sum/2  "Crmbeta"
  Crmrde/1(Crmrde) -> Sum/18  "Crmrde"

== system aerotest/RollMomentCoefficient/MachRegion3 ==
  note: 0.5 <= Mach <= 1.4
  AeroIn_Bus : Inport
  Bus Creator : BusCreator  Inputs=3
  Crmbasic : Subsystem
  Crmbde : Subsystem
  Crmbdle : Subsystem
  Crmbdn : Subsystem
  Crmbeta : Subsystem
  Crmbetad : Subsystem
  Crmblg : Subsystem
  Crmdai : Subsystem
  Crmdaib : Subsystem
  Crmday : Subsystem
  Crmdayb : Subsystem
  Crmdna : Subsystem
  Crmdr : Subsystem
  Crmp : Subsystem
  Crmpbeta : Subsystem
  Crmr : Subsystem
  Crmrbeta : Subsystem
  Crmrde : Subsystem
  Sum : Sum  Inputs=18
  eoeff1 : Subsystem
  crmtot : Outport
  wires:
  Sum/1 -> crmtot/1
  Crmrde/1(Crmrde) -> Sum/18  "Crmrde"
  Crmrbeta/1(Crmrbeta) -> Sum/17  "Crmrbeta"
  Crmr/1(Crmr) -> Sum/16  "Crmr"
  Crmpbeta/1(Crmpbeta) -> Sum/15  "Crmpbeta"
  Crmp/1(Crmp) -> Sum/14  "Crmp"
  Crmbetad/1(Crmbetad) -> Sum/13  "Crmbetad"
  Crmdna/1(Crmdna) -> Sum/12  "Crmdna"
  Crmdayb/1(Crmdayb) -> Sum/11  "Crmdayb"
  Crmday/1(Crmday) -> Sum/10  "Crmday"
  Crmdaib/1(Crmdaib) -> Sum/9  "Crmdaib"
  Crmdai/1(Crmdai) -> Sum/8  "Crmdai"
  Crmdr/1(Crmdr) -> Sum/7  "Crmdr"
  Crmblg/1(Crmblg) -> Sum/6  "Crmblg"
  Crmbdle/1(Crmbdle) -> Sum/5  "Crmbdle"
  Crmbdn/1(Crmbdn) -> Sum/4  "Crmbdn"
  Crmbde/1(Crmbde) -> Sum/3  "Crmbde"
  Crmbeta/1(Crmbeta) -> Sum/2  "Crmbeta"
  Crmbasic/1(Crmbasic) -> Sum/1  "Crmbasic"
  eoeff1/2(eieff) -> Bus Creator/3  "eieff"
  eoeff1/1(eoeff) -> Bus Creator/2  "eoeff"
  Bus Creator/1 -> Crmr/1(in_bus), Crmrde/1(in_bus), Crmp/1(in_bus), Crmbetad/1(in_bus), Crmdna/1(in_bus), Crmday/1(in_bus), Crmdai/1(in_bus), Crmdr/1(in_bus), Crmblg/1(in_bus), Crmbdle/1(in_bus), Crmbdn/1(in_bus), Crmbde/1(in_bus), Crmbeta/1(in_bus)  "in_bus"
  AeroIn_Bus/1 -> eoeff1/1(AeroIn_Bus), Bus Creator/1

== system aerotest/RollMomentCoefficient/MachRegion4 ==
  note: 1.4 < Mach
  AeroIn_Bus : Inport
  Bus Creator : BusCreator  Inputs=3
  Crmbasic : Subsystem
  Crmbde : Subsystem
  Crmbdle : Subsystem
  Crmbdn : Subsystem
  Crmbeta : Subsystem
  Crmbetad : Subsystem
  Crmblg : Subsystem
  Crmdai : Subsystem
  Crmdaib : Subsystem
  Crmday : Subsystem
  Crmdayb : Subsystem
  Crmdna : Subsystem
  Crmdr : Subsystem
  Crmp : Subsystem
  Crmpbeta : Subsystem
  Crmr : Subsystem
  Crmrbeta : Subsystem
  Crmrde : Subsystem
  Sum : Sum  Inputs=18
  eoeff1 : Subsystem
  crmtot : Outport
  wires:
  Crmrde/1(Crmrde) -> Sum/18  "Crmrde"
  Crmrbeta/1(Crmrbeta) -> Sum/17  "Crmrbeta"
  Crmr/1(Crmr) -> Sum/16  "Crmr"
  Crmpbeta/1(Crmpbeta) -> Sum/15  "Crmpbeta"
  Crmp/1(Crmp) -> Sum/14  "Crmp"
  Crmbetad/1(Crmbetad) -> Sum/13  "Crmbetad"
  Crmdna/1(Crmdna) -> Sum/12  "Crmdna"
  Crmdayb/1(Crmdayb) -> Sum/11  "Crmdayb"
  Crmday/1(Crmday) -> Sum/10  "Crmday"
  Crmdaib/1(Crmdaib) -> Sum/9  "Crmdaib"
  Crmdai/1(Crmdai) -> Sum/8  "Crmdai"
  Crmdr/1(Crmdr) -> Sum/7  "Crmdr"
  Crmblg/1(Crmblg) -> Sum/6  "Crmblg"
  Crmbdle/1(Crmbdle) -> Sum/5  "Crmbdle"
  Crmbdn/1(Crmbdn) -> Sum/4  "Crmbdn"
  Crmbde/1(Crmbde) -> Sum/3  "Crmbde"
  Crmbeta/1(Crmbeta) -> Sum/2  "Crmbeta"
  Crmbasic/1(Crmbasic) -> Sum/1  "Crmbasic"
  eoeff1/1(eoeff) -> Bus Creator/2  "eoeff"
  AeroIn_Bus/1 -> eoeff1/1(AeroIn_Bus), Bus Creator/1
  Bus Creator/1 -> Crmr/1(in_bus), Crmrde/1(in_bus), Crmp/1(in_bus), Crmbetad/1(in_bus), Crmdna/1(in_bus), Crmday/1(in_bus), Crmdai/1(in_bus), Crmdr/1(in_bus), Crmblg/1(in_bus), Crmbdle/1(in_bus), Crmbdn/1(in_bus), Crmbde/1(in_bus), Crmbeta/1(in_bus)  "in_bus"
  eoeff1/2(eieff) -> Bus Creator/3  "eieff"
  Sum/1 -> crmtot/1

== system aerotest/RollMomentCoefficient/Subsystem ==
  mach_nd : Inport
  CrmtotMR1 : Inport  Port=2
  CrmtotMR2 : Inport  Port=3
  CrmtotMR3 : Inport  Port=4
  CrmtotMR4 : Inport  Port=5
  AND : Logic  IconShape=distinctive  AllPortsSameDT=off  OutDataTypeStr=boolean
  AND1 : Logic  IconShape=distinctive  AllPortsSameDT=off  OutDataTypeStr=boolean
  Compare To Constant1 : simulink/Logic and Bit Operations/Compare To Constant  relop=<=  const=0.4  OutDataTypeStr=boolean
  Compare To Constant2 : simulink/Logic and Bit Operations/Compare To Constant  relop=>  const=0.4  OutDataTypeStr=boolean
  Compare To Constant3 : simulink/Logic and Bit Operations/Compare To Constant  relop=<  const=0.5  OutDataTypeStr=boolean
  Compare To Constant4 : simulink/Logic and Bit Operations/Compare To Constant  relop=<=  const=1.4  OutDataTypeStr=boolean
  Compare To Constant5 : simulink/Logic and Bit Operations/Compare To Constant  relop=>=  const=0.5  OutDataTypeStr=boolean
  Switch : Switch  Criteria=u2 ~= 0
  Switch1 : Switch  Criteria=u2 ~= 0
  Switch2 : Switch  Criteria=u2 ~= 0
  Crmtot : Outport
  wires:
  Compare To Constant5/1 -> AND1/1
  Compare To Constant4/1 -> AND1/2
  AND1/1 -> Switch2/2
  CrmtotMR4/1 -> Switch2/3
  CrmtotMR3/1 -> Switch2/1
  Switch/1 -> Crmtot/1
  Switch2/1 -> Switch1/3
  CrmtotMR2/1 -> Switch1/1
  Switch1/1 -> Switch/3
  CrmtotMR1/1 -> Switch/1
  AND/1 -> Switch1/2
  Compare To Constant3/1 -> AND/2
  Compare To Constant2/1 -> AND/1
  Compare To Constant1/1 -> Switch/2
  mach_nd/1 -> Compare To Constant1/1, Compare To Constant3/1, Compare To Constant4/1, Compare To Constant5/1, Compare To Constant2/1

== system aerotest/TangentialForceCoefficient/MachRegion1 ==
  note: Mach <= 0.4
  AeroIn_Bus : Inport
  Bus Creator : BusCreator  Inputs=3
  Ctalfa : Subsystem
  Ctbasic : Subsystem
  Ctbeta : Subsystem
  Ctda : Subsystem
  Ctdedn : Subsystem
  Ctdei : Subsystem
  Ctdey : Subsystem
  Ctdle : Subsystem
  Ctdn : Subsystem
  Ctdr : Subsystem
  Cthigh : Subsystem
  Ctlg : Subsystem
  Sum : Sum  Inputs=12
  eoeff : Subsystem
  cttotMR1 : Outport
  wires:
  Ctdedn/1(Ctdedn) -> Sum/5  "Ctdedn"
  Ctdey/1(Ctdey) -> Sum/4  "Ctdey"
  Ctdei/1(Ctdei) -> Sum/3  "Ctdei"
  Ctalfa/1(Ctalfa) -> Sum/2  "Ctalfa"
  Ctbasic/1(Ctbasic) -> Sum/1  "Ctbasic"
  Cthigh/1(Cthigh) -> Sum/12  "Cthigh"
  Ctdr/1(Ctdr) -> Sum/11  "Ctdr"
  Ctda/1(Ctda) -> Sum/10  "Ctda"
  Ctbeta/1(Ctbeta) -> Sum/9  "Ctbeta"
  Ctlg/1(Ctlg) -> Sum/8  "Ctlg"
  Ctdle/1(Ctdle) -> Sum/7  "Ctdle"
  Ctdn/1(Ctdn) -> Sum/6  "Ctdn"
  Bus Creator/1 -> Ctbasic/1(in_bus), Ctalfa/1(in_bus), Ctdei/1(in_bus), Ctdey/1(in_bus), Ctdedn/1(in_bus), Ctdn/1(in_bus), Ctdle/1(in_bus), Ctlg/1(in_bus), Ctbeta/1(in_bus), Ctda/1(in_bus), Ctdr/1(in_bus), Cthigh/1(in_bus)  "in_bus"
  eoeff/2(eieff) -> Bus Creator/3  "eieff"
  eoeff/1(eoeff) -> Bus Creator/2  "eoeff"
  AeroIn_Bus/1 -> Bus Creator/1, eoeff/1(AeroIn_Bus)
  Sum/1 -> cttotMR1/1

== system aerotest/TangentialForceCoefficient/MachRegion2 ==
  note: 0.4 < Mach < 0.5
  AeroIn_Bus : Inport
  Bus Creator : BusCreator  Inputs=5
  Ctalfa : Subsystem
  Ctbasic : Subsystem
  Ctbeta : Subsystem
  Ctda : Subsystem
  Ctdedn : Subsystem
  Ctdei : Subsystem
  Ctdey : Subsystem
  Ctdle : Subsystem
  Ctdn : Subsystem
  Ctdr : Subsystem
  Cthigh : Subsystem
  Ctlg : Subsystem
  Sum : Sum  Inputs=12
  eoeff : Subsystem
  cttotMR2 : Outport
  wires:
  Cthigh/1(Cthigh) -> Sum/12  "Cthigh"
  Ctdr/1(Ctdr) -> Sum/11  "Ctdr"
  Ctda/1(Ctda) -> Sum/10  "Ctda"
  Ctbeta/1(Ctbeta) -> Sum/9  "Ctbeta"
  Ctlg/1(Ctlg) -> Sum/8  "Ctlg"
  Ctdle/1(Ctdle) -> Sum/7  "Ctdle"
  Ctdn/1(Ctdn) -> Sum/6  "Ctdn"
  eoeff/4(eieffhigh) -> Bus Creator/5  "eieffhigh"
  eoeff/3(eoeffhigh) -> Bus Creator/4  "eoeffhigh"
  Sum/1 -> cttotMR2/1
  AeroIn_Bus/1 -> Bus Creator/1
  eoeff/1(eoefflow) -> Bus Creator/2  "eoefflow"
  eoeff/2(eiefflow) -> Bus Creator/3  "eiefflow"
  Bus Creator/1 -> Ctdr/1(in_bus), Ctda/1(in_bus), Ctbeta/1(in_bus), Ctlg/1(in_bus), Ctdle/1(in_bus), Ctdn/1(in_bus), Ctdedn/1(in_bus), Ctdey/1(in_bus), Ctdei/1(in_bus), Ctalfa/1(in_bus), Ctbasic/1(in_bus)  "in_bus"
  Ctdei/1(Ctdei) -> Sum/3  "Ctdei"
  Ctalfa/1(Ctalfa) -> Sum/2  "Ctalfa"
  Ctdey/1(Ctdey) -> Sum/4  "Ctdey"
  Ctbasic/1(Ctbasic) -> Sum/1  "Ctbasic"
  Ctdedn/1(Ctdedn) -> Sum/5  "Ctdedn"

== system aerotest/TangentialForceCoefficient/MachRegion3 ==
  note: 0.5 < Mach
  AeroIn_Bus : Inport
  Bus Creator : BusCreator  Inputs=3
  Ctalfa : Subsystem
  Ctbasic : Subsystem
  Ctbeta : Subsystem
  Ctda : Subsystem
  Ctdedn : Subsystem
  Ctdei : Subsystem
  Ctdey : Subsystem
  Ctdle : Subsystem
  Ctdn : Subsystem
  Ctdr : Subsystem
  Cthigh : Subsystem
  Ctlg : Subsystem
  Sum : Sum  Inputs=12
  eoeff : Subsystem
  cttotMR3 : Outport
  wires:
  eoeff/2(eieff) -> Bus Creator/3  "eieff"
  eoeff/1(eoeff) -> Bus Creator/2  "eoeff"
  Cthigh/1(Cthigh) -> Sum/12  "Cthigh"
  Ctdr/1(Ctdr) -> Sum/11  "Ctdr"
  Ctda/1(Ctda) -> Sum/10  "Ctda"
  Ctbeta/1(Ctbeta) -> Sum/9  "Ctbeta"
  Ctlg/1(Ctlg) -> Sum/8  "Ctlg"
  Ctdle/1(Ctdle) -> Sum/7  "Ctdle"
  Ctdn/1(Ctdn) -> Sum/6  "Ctdn"
  Ctdedn/1(Ctdedn) -> Sum/5  "Ctdedn"
  Ctbasic/1(Ctbasic) -> Sum/1  "Ctbasic"
  Ctdey/1(Ctdey) -> Sum/4  "Ctdey"
  Ctalfa/1(Ctalfa) -> Sum/2  "Ctalfa"
  Ctdei/1(Ctdei) -> Sum/3  "Ctdei"
  Bus Creator/1 -> Ctbasic/1(in_bus), Ctalfa/1(in_bus), Ctdei/1(in_bus), Ctdn/1(in_bus), Ctdle/1(in_bus), Ctlg/1(in_bus), Ctda/1(in_bus), Ctdr/1(in_bus), Ctdey/1(in_bus)  "in_bus"
  AeroIn_Bus/1 -> eoeff/1(AeroIn_Bus), Bus Creator/1
  Sum/1 -> cttotMR3/1

== system aerotest/TangentialForceCoefficient/Subsystem ==
  mach_nd : Inport
  cttotMR1 : Inport  Port=2
  cttotMR2 : Inport  Port=3
  cttotMR3 : Inport  Port=4
  AND : Logic  IconShape=distinctive  AllPortsSameDT=off  OutDataTypeStr=boolean
  Compare To Constant1 : simulink/Logic and Bit Operations/Compare To Constant  relop=<=  const=0.4  OutDataTypeStr=boolean
  Compare To Constant2 : simulink/Logic and Bit Operations/Compare To Constant  relop=>  const=0.4  OutDataTypeStr=boolean
  Compare To Constant3 : simulink/Logic and Bit Operations/Compare To Constant  relop=<  const=0.5  OutDataTypeStr=boolean
  Switch : Switch  Criteria=u2 ~= 0
  Switch1 : Switch  Criteria=u2 ~= 0
  Out1 : Outport
  wires:
  Switch/1 -> Out1/1
  cttotMR3/1 -> Switch1/3
  cttotMR2/1 -> Switch1/1
  Switch1/1 -> Switch/3
  cttotMR1/1 -> Switch/1
  AND/1 -> Switch1/2
  Compare To Constant3/1 -> AND/2
  Compare To Constant2/1 -> AND/1
  Compare To Constant1/1 -> Switch/2
  mach_nd/1 -> Compare To Constant1/1, Compare To Constant3/1, Compare To Constant2/1

== system aerotest/YawMomentCoefficient/MachRegion1 ==
  note: Mach <= 0.4
  AeroIn_Bus : Inport
  Bus Creator : BusCreator  Inputs=3
  Cymbasic : Subsystem
  Cymbcai : Subsystem
  Cymbde : Subsystem
  Cymbdle : Subsystem
  Cymbdn : Subsystem
  Cymbeta : Subsystem
  Cymbetad : Subsystem
  Cymblg : Subsystem
  Cymdai : Subsystem
  Cymdaib : Subsystem
  Cymday : Subsystem
  Cymdayb : Subsystem
  Cymdna : Subsystem
  Cymdr : Subsystem
  Cymp : Subsystem
  Cympbeta : Subsystem
  Cymr : Subsystem
  Cymrbeta : Subsystem
  Sum : Sum  Inputs=18
  eoeff : Subsystem
  Cymtot : Outport
  wires:
  Cymbasic/1(Cymbasic) -> Sum/1  "Cymbasic"
  Cymbdn/1(Cymbdn) -> Sum/4  "Cymbdn"
  Cymbeta/1(Cymbeta) -> Sum/2  "Cymbeta"
  Cymbetad/1(Cymbetad) -> Sum/14  "Cymbetad"
  Cymday/1(Cymday) -> Sum/11  "Cymday"
  Cymp/1(Cymp) -> Sum/15  "Cymp"
  Cymdna/1(Cymdna) -> Sum/13  "Cymdna"
  eoeff/1(eoeff) -> Bus Creator/2  "eoeff"
  Cymr/1(Cymr) -> Sum/17  "Cymr"
  AeroIn_Bus/1 -> eoeff/1(AeroIn_Bus), Bus Creator/1
  Cymbde/1(Cymbde) -> Sum/3  "Cymbde"
  Cymbcai/1(Cymbcai) -> Sum/6  "Cymbcai"
  Cymblg/1(Cymblg) -> Sum/7  "Cymblg"
  Cymdaib/1(Cymdaib) -> Sum/10  "Cymdaib"
  Cymdai/1(Cymdai) -> Sum/9  "Cymdai"
  Cymdr/1(Cymdr) -> Sum/8  "Cymdr"
  Cymrbeta/1(Cymrbeta) -> Sum/18  "Cymrbeta"
  Bus Creator/1 -> Cympbeta/1(in_bus), Cymr/1(in_bus), Cymrbeta/1(in_bus), Cymp/1(in_bus), Cymbetad/1(in_bus), Cymdna/1(in_bus), Cymdayb/1(in_bus), Cymday/1(in_bus), Cymdaib/1(in_bus), Cymdai/1(in_bus), Cymdr/1(in_bus), Cymblg/1(in_bus), Cymbcai/1(in_bus), Cymbdle/1(in_bus), Cymbdn/1(in_bus), Cymbde/1(in_bus), Cymbeta/1(in_bus), Cymbasic/1(in_bus)  "in_bus"
  Cymdayb/1(Cymdayb) -> Sum/12  "Cymdayb"
  Cympbeta/1(Cympbeta) -> Sum/16  "Cympbeta"
  Cymbdle/1(Cymbdle) -> Sum/5  "Cymbdle"
  eoeff/2(eieff) -> Bus Creator/3  "eieff"
  Sum/1 -> Cymtot/1

== system aerotest/YawMomentCoefficient/MachRegion2 ==
  note: 0.4 < Mach < 0.5
  AeroIn_Bus : Inport
  Bus Creator : BusCreator  Inputs=3
  Cymbasic : Subsystem
  Cymbcai : Subsystem
  Cymbde : Subsystem
  Cymbdle : Subsystem
  Cymbdn : Subsystem
  Cymbeta : Subsystem
  Cymbetad : Subsystem
  Cymblg : Subsystem
  Cymdai : Subsystem
  Cymdaib : Subsystem
  Cymday : Subsystem
  Cymdayb : Subsystem
  Cymdna : Subsystem
  Cymdr : Subsystem
  Cymp : Subsystem
  Cympbeta : Subsystem
  Cymr : Subsystem
  Cymrbeta : Subsystem
  Sum : Sum  Inputs=18
  eoeff : Subsystem
  Cymtot : Outport
  wires:
  Cympbeta/1(Cympbeta) -> Sum/16  "Cympbeta"
  eoeff/2(eieff) -> Bus Creator/3  "eieff"
  Cymdaib/1(Cymdaib) -> Sum/10  "Cymdaib"
  Cymbdle/1(Cymbdle) -> Sum/5  "Cymbdle"
  Cymdr/1(Cymdr) -> Sum/8  "Cymdr"
  Cymr/1(Cymr) -> Sum/17  "Cymr"
  Cymdayb/1(Cymdayb) -> Sum/12  "Cymdayb"
  Cymdai/1(Cymdai) -> Sum/9  "Cymdai"
  Cymrbeta/1(Cymrbeta) -> Sum/18  "Cymrbeta"
  Bus Creator/1 -> Cympbeta/1(in_bus), Cymr/1(in_bus), Cymrbeta/1(in_bus), Cymp/1(in_bus), Cymbetad/1(in_bus), Cymdna/1(in_bus), Cymdayb/1(in_bus), Cymday/1(in_bus), Cymdaib/1(in_bus), Cymdai/1(in_bus), Cymdr/1(in_bus), Cymblg/1(in_bus), Cymbcai/1(in_bus), Cymbdle/1(in_bus), Cymbdn/1(in_bus), Cymbde/1(in_bus), Cymbeta/1(in_bus), Cymbasic/1(in_bus)  "in_bus"
  eoeff/1(eoeff) -> Bus Creator/2  "eoeff"
  Cymbasic/1(Cymbasic) -> Sum/1  "Cymbasic"
  Cymblg/1(Cymblg) -> Sum/7  "Cymblg"
  Cymbde/1(Cymbde) -> Sum/3  "Cymbde"
  AeroIn_Bus/1 -> eoeff/1(AeroIn_Bus), Bus Creator/1
  Cymbcai/1(Cymbcai) -> Sum/6  "Cymbcai"
  Cymbeta/1(Cymbeta) -> Sum/2  "Cymbeta"
  Cymbdn/1(Cymbdn) -> Sum/4  "Cymbdn"
  Cymp/1(Cymp) -> Sum/15  "Cymp"
  Cymbetad/1(Cymbetad) -> Sum/14  "Cymbetad"
  Cymday/1(Cymday) -> Sum/11  "Cymday"
  Cymdna/1(Cymdna) -> Sum/13  "Cymdna"
  Sum/1 -> Cymtot/1

== system aerotest/YawMomentCoefficient/MachRegion3 ==
  note: 0.5 <= Mach <= 1.4
  AeroIn_Bus : Inport
  Bus Creator : BusCreator  Inputs=3
  Cymbasic : Subsystem
  Cymbcai : Subsystem
  Cymbde : Subsystem
  Cymbdle : Subsystem
  Cymbdn : Subsystem
  Cymbeta : Subsystem
  Cymbetad : Subsystem
  Cymblg : Subsystem
  Cymdai : Subsystem
  Cymdaib : Subsystem
  Cymday : Subsystem
  Cymdayb : Subsystem
  Cymdna : Subsystem
  Cymdr : Subsystem
  Cymp : Subsystem
  Cympbeta : Subsystem
  Cymr : Subsystem
  Cymrbeta : Subsystem
  Sum : Sum  Inputs=18
  eoeff : Subsystem
  Cymtot : Outport
  wires:
  Cymbasic/1(Cymbasic) -> Sum/1  "Cymbasic"
  Cymp/1(Cymp) -> Sum/15  "Cymp"
  Cymday/1(Cymday) -> Sum/11  "Cymday"
  AeroIn_Bus/1 -> eoeff/1(AeroIn_Bus), Bus Creator/1
  Cympbeta/1(Cympbeta) -> Sum/16  "Cympbeta"
  Cymbde/1(Cymbde) -> Sum/3  "Cymbde"
  Cymdna/1(Cymdna) -> Sum/13  "Cymdna"
  Cymbdn/1(Cymbdn) -> Sum/4  "Cymbdn"
  Bus Creator/1 -> Cymr/1(in_bus), Cymp/1(in_bus), Cymbetad/1(in_bus), Cymdna/1(in_bus), Cymday/1(in_bus), Cymdai/1(in_bus), Cymdr/1(in_bus), Cymblg/1(in_bus), Cymbcai/1(in_bus), Cymbdle/1(in_bus), Cymbdn/1(in_bus), Cymbde/1(in_bus), Cymbeta/1(in_bus)  "in_bus"
  eoeff/2(eieff) -> Bus Creator/3  "eieff"
  Cymdaib/1(Cymdaib) -> Sum/10  "Cymdaib"
  Cymblg/1(Cymblg) -> Sum/7  "Cymblg"
  eoeff/1(eoeff) -> Bus Creator/2  "eoeff"
  Cymdayb/1(Cymdayb) -> Sum/12  "Cymdayb"
  Cymbdle/1(Cymbdle) -> Sum/5  "Cymbdle"
  Cymdr/1(Cymdr) -> Sum/8  "Cymdr"
  Cymdai/1(Cymdai) -> Sum/9  "Cymdai"
  Cymr/1(Cymr) -> Sum/17  "Cymr"
  Cymbetad/1(Cymbetad) -> Sum/14  "Cymbetad"
  Cymbcai/1(Cymbcai) -> Sum/6  "Cymbcai"
  Cymrbeta/1(Cymrbeta) -> Sum/18  "Cymrbeta"
  Cymbeta/1(Cymbeta) -> Sum/2  "Cymbeta"
  Sum/1 -> Cymtot/1

== system aerotest/YawMomentCoefficient/MachRegion4 ==
  note: 1.4 < Mach
  AeroIn_Bus : Inport
  Bus Creator : BusCreator  Inputs=3
  Cymbasic : Subsystem
  Cymbcai : Subsystem
  Cymbde : Subsystem
  Cymbdle : Subsystem
  Cymbdn : Subsystem
  Cymbeta : Subsystem
  Cymbetad : Subsystem
  Cymblg : Subsystem
  Cymdai : Subsystem
  Cymdaib : Subsystem
  Cymday : Subsystem
  Cymdayb : Subsystem
  Cymdna : Subsystem
  Cymdr : Subsystem
  Cymp : Subsystem
  Cympbeta : Subsystem
  Cymr : Subsystem
  Cymrbeta : Subsystem
  Sum : Sum  Inputs=18
  eoeff : Subsystem
  Cymtot : Outport
  wires:
  Sum/1 -> Cymtot/1
  Cymbeta/1(Cymbeta) -> Sum/2  "Cymbeta"
  Cymrbeta/1(Cymrbeta) -> Sum/18  "Cymrbeta"
  Cymbcai/1(Cymbcai) -> Sum/6  "Cymbcai"
  Cymbetad/1(Cymbetad) -> Sum/14  "Cymbetad"
  Cymr/1(Cymr) -> Sum/17  "Cymr"
  Cymdai/1(Cymdai) -> Sum/9  "Cymdai"
  Cymdr/1(Cymdr) -> Sum/8  "Cymdr"
  Cymbdle/1(Cymbdle) -> Sum/5  "Cymbdle"
  Cymdayb/1(Cymdayb) -> Sum/12  "Cymdayb"
  eoeff/1(eoeff) -> Bus Creator/2  "eoeff"
  Cymblg/1(Cymblg) -> Sum/7  "Cymblg"
  Cymdaib/1(Cymdaib) -> Sum/10  "Cymdaib"
  eoeff/2(eieff) -> Bus Creator/3  "eieff"
  Bus Creator/1 -> Cymbeta/1(in_bus), Cymbde/1(in_bus), Cymbdn/1(in_bus), Cymbdle/1(in_bus), Cymbcai/1(in_bus), Cymblg/1(in_bus), Cymdr/1(in_bus), Cymdai/1(in_bus), Cymday/1(in_bus), Cymdna/1(in_bus), Cymbetad/1(in_bus), Cymp/1(in_bus), Cymr/1(in_bus)  "in_bus"
  Cymbdn/1(Cymbdn) -> Sum/4  "Cymbdn"
  Cymdna/1(Cymdna) -> Sum/13  "Cymdna"
  Cymbde/1(Cymbde) -> Sum/3  "Cymbde"
  Cympbeta/1(Cympbeta) -> Sum/16  "Cympbeta"
  AeroIn_Bus/1 -> Bus Creator/1, eoeff/1(AeroIn_Bus)
  Cymday/1(Cymday) -> Sum/11  "Cymday"
  Cymp/1(Cymp) -> Sum/15  "Cymp"
  Cymbasic/1(Cymbasic) -> Sum/1  "Cymbasic"
